simulink model "lab3_ssEvals"  (R2024b)
settings: Solver=VariableStepAuto  StartTime=0.0  StopTime=sIn.simulation_time  RelTol=1e-3
undefined symbols (not defined in the file or in its folder): feedback, filt, sens
libraries: simulink x1
settings Model: Creator=pries  LastModifiedBy=pries
settings DataIOCC: ReturnWorkspaceOutputs=off

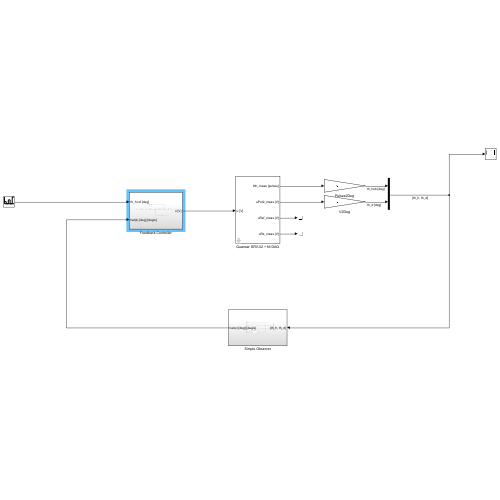
[thumbnail: Simulink's stored preview of the top-level diagram]
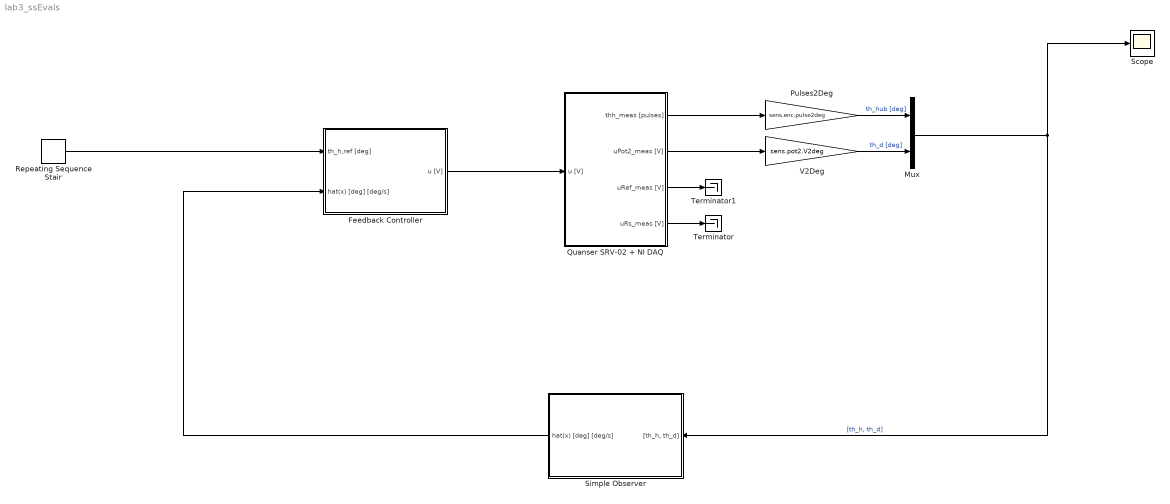
== system lab3_ssEvals ==
  Feedback Controller : Subsystem
  Mux : Mux  Inputs=2
  Pulses2Deg : Gain  Gain=sens.enc.pulse2deg
  Quanser SRV-02 + NI DAQ : Subsystem  mask(Quanser SRV-02 (with resonant load) + NI DAQ){Ts=0.001, fricType=Coulomb + viscous, lockShaft=off, beamInitPos=10}
      mask prompts: Ts "NI DAQ Sample Time:"; fricType "Friction model"; lockShaft "Lock motor shaft"; beamInitPos "Beam initial position [deg]:"
      mask help: Quanser SRV-02 (with resonant load) + NI DAQ model.
      mask init:
      | %%
      | % Riccardo Antonello (riccardo.antonello@unipd.it)
      | %
      | % April 28, 2020
      | %
      | % Dept. of Information Engineering, University of Padova
      | %
      | 
      | %%  Conversion gains
      | deg2rad = pi/180;                   %   [deg]   -> [rad]
      | rad2deg = 180/pi;                   %   [rad]   -> [deg]
      | 
      | 
      | %%  Sensors data
      | 
      | %   shunt resistor
      | sens.curr.Rs = 0.5;   
      | 
      | %   Hewlett-Packard HEDS-5540#A06 optical encoder
      | sens.enc.ppr = 500*4;                                                   %   pulses per rotation
      | sens.enc.pulse2deg = 360/sens.enc.ppr;                                  %   [pulses] -> [deg]
      | sens.enc.pulse2rad = 2*pi/sens.enc.ppr;                                 %   [pulses] -> [rad]
      | sens.enc.deg2pulse = sens.enc.ppr/360;                                  %   [deg] -> [pulses]
      | sens.enc.rad2pulse = sens.enc.ppr/2/pi;                                 %   [rad] -> [pulses]
      | 
      | %   potentiometer 2 (Spectrol 357-0-0-103) - installed on hub
      | sens.pot2.range.R      = 10e3;                                          %   ohmic value range 
      | sens.pot2.range.V      = 5;                                             %   voltage range
      | sens.pot2.range.th_deg = 340;                                           %   angle range [deg]
      | sens.pot2.range.th     = sens.pot2.range.th_deg * deg2rad;              %   angle range [rad]                           
      | sens.pot2.deg2V        = sens.pot2.range.V / sens.pot2.range.th_deg;    %   sensitivity [V/deg]
      | sens.pot2.rad2V        = sens.pot2.range.V / sens.pot2.range.th;        %   sensitivity [V/rad]
      | sens.pot2.V2deg        = 1/sens.pot2.deg2V;                             %   conversion gain [V] -> [deg]
      | sens.pot2.V2rad        = 1/sens.pot2.rad2V;                             %   conversion gain [V] -> [rad]
      | sens.pot2.noise.var    = 3.5e-7;                                        %   out noise variance [V^2]
      | 
      | 
      | %%  Data acquisition board (daq) data
      | 
      | %   NI PCI-6221 DAC data
      | daq.dac.bits = 16;                                  %   resolution (bits)
      | daq.dac.fs   = 10;                                  %   full scale 
      | daq.dac.q    = 2*daq.dac.fs/(2^daq.dac.bits-1);     %	quantization
      | 
      | %   NI PCI-6221 ADC data
      | daq.adc.bits = 16;                                  %   resolution (bits)
      | daq.adc.fs   = 10;                                  %   full scale (as set in SLDRT Analog Input block)
      | daq.adc.q    = 2*daq.adc.fs/(2^daq.adc.bits-1);     %   quantization   
      | 
      | 
      | %%  Set beam initial position
      | % SRV02Handle = find_system(gcb, ...
      | %     'LookUnderMasks', 'on', ...
      | %     'FindAll', 'on', ...
      | %     'FollowLinks', 'on', ...
      | %     'SearchDepth', '1', ...
      | %     'BlockType', 'ModelReference', ...
      | %     'Name', 'Quanser SRV-02');
      | %
      | % %get_param(SRV02Handle, 'InstanceParameters')
      | % InstanceParams = get_param(SRV02Handle, 'InstanceParameters');
      | % for k = 1:length(InstanceParams)
      | %     if strcmp(InstanceParams(k).Name, 'thb0')
      | %         if lockShaft
      | %             InstanceParams(k).Value = sprintf('%f', beamInitPos);
      | %         else
      | %             InstanceParams(k).Value = sprintf('%f', 0);    
      | %         end
      | %         set_param(SRV02Handle, 'InstanceParameters', InstanceParams);
      | %         break;
      | %     end
      | % end
      | 
      | if lockShaft
      |     thb0 = beamInitPos;
      | else
      |     thb0 = 0;    
      | end
      | 
      | 
      | %%  Mask initialization
      | if lockShaft
      |     
      |     %   find Inport handle
      |     InPortHandle = find_system(gcb, ...
      |         'LookUnderMasks', 'on', ...
      |         'FindAll', 'on', ...
      |         'FollowLinks', 'on', ...
      |         'SearchDepth', '1', ...
      |         'BlockType', 'Inport', ...
      |         'Name', 'u [V]');
      |     
      |     if ~isempty(InPortHandle)
      |     
      |         %   find DAC handle
      |         DACHandle = find_system(gcb, ...
      |             'LookUnderMasks', 'on', ...
      |             'FindAll', 'on', ...
      |             'FollowLinks', 'on', ...
      |             'SearchDepth', '1', ...
      |             'BlockType', 'SubSystem', ...
      |             'Name', 'DAC');  
      | 
      |         %   remove Inport output connection   
      |         InportConn = get_param(InPortHandle, 'PortConnectivity');
      |         delete_line(gcb, InportConn.Position);
      | 
      |         %   remove Inport block
      |         delete_block(InPortHandle);
      | 
      |         %   add Constant block
      |         ConstantHandle = add_block( ...
      |             'simulink/Sources/Constant', [gcb, '/u [V]'], ...
      |             'Position', [20   -37    50   -23], ...
      |             'Value', '0');
      | 
      |         %   connect Constant to DAC block
      |         DACPortHandles = get_param(DACHandle, 'PortHandles');
      |         ConstantPortHandles = get_param(ConstantHandle, 'PortHandles');
      |         add_line(gcb, ConstantPortHandles.Outport(1), DACPortHandles.Inport(1));
      |     
      |     end
      |     
      | else
      |     
      |     %   find Constant handle
      |     ConstantHandle = find_system(gcb, ...
      |         'LookUnderMasks', 'on', ...
      |         'FindAll', 'on', ...
      |         'FollowLinks', 'on', ...
      |         'SearchDepth', '1', ...
      |         'BlockType', 'Constant', ...
      |         'Name', 'u [V]');
      |     
      |     if ~isempty(ConstantHandle)
      |     
      |         %   find DAC handle
      |         DACHandle = find_system(gcb, ...
      |             'LookUnderMasks', 'on', ...
      |             'FindAll', 'on', ...
      |             'FollowLinks', 'on', ...
      |             'SearchDepth', '1', ...
      |             'BlockType', 'SubSystem', ...
      |             'Name', 'DAC');  
      |  
      |         %   remove Constant output connection   
      |         ConstantConn = get_param(ConstantHandle, 'PortConnectivity');
      |         delete_line(gcb, ConstantConn.Position);
      | 
      |         %   remove Inport block
      |         delete_block(ConstantHandle);   
      | 
      |         %   add Inport block
      |         InportHandle = add_block( ...
      |             'simulink/Sources/In1', [gcb, '/u [V]'], ...
      |             'Position', [20   -37    50   -23], ...
      |             'Port', '1');
      | 
      |         %   connect Constant to DAC block
      |         DACPortHandles = get_param(DACHandle, 'PortHandles');
      |         InportPortHandles = get_param(InportHandle, 'PortHandles');
      |         add_line(gcb, InportPortHandles.Outport(1), DACPortHandles.Inport(1));
      |     
      |      end
      |     
      | end
      mask Help:
      | Riccardo Antonello (antonello@dei.unipd.it)
      | 
      | April 28, 2020
      | 
      | Dept. of Information Engineering, University of Padova
      mask TypeOptions fricType: Coulomb + viscous | Karnopp
      mask Callback lockShaft:
      | %   get status of check box
      | lockShaft = get_param(gcb, 'lockShaft');
      | 
      | %   get current value of MaskVisibilities property
      | maskVisibilities = get_param(gcb, 'MaskVisibilities');
      | 
      | %   set visibility of the dialog box element
      | if strcmp(lockShaft, 'on')
      |     maskVisibilities{4} = 'on';
      | else
      |     maskVisibilities{4} = 'off';
      | end
      | 
      | % Set the 'MaskVisibilities' property for each parameter in mask
      | set_param( gcb, 'MaskVisibilities', maskVisibilities);
  Repeating Sequence Stair : simulink/Sources/Repeating Sequence Stair  OutValues=sIn.position  tsamp=sIn.step_time  OutMin=[]  OutMax=[]  OutDataTypeStr=double  OutputDataTypeScalingMode=double  OutDataType=fixdt(0,8)  ConRadixGroup=Best Precision: Vector-wise  OutScaling=2^-12
  Scope : Scope
  Simple Observer : Subsystem
  Terminator : Terminator
  Terminator1 : Terminator
  V2Deg : Gain  Gain=sens.pot2.V2deg
  wires:
  Quanser SRV-02 + NI DAQ/1(thh_meas [pulses]) -> Pulses2Deg/1
  Quanser SRV-02 + NI DAQ/2(uPot2_meas [V]) -> V2Deg/1
  Quanser SRV-02 + NI DAQ/4(uRs_meas [V]) -> Terminator/1
  Quanser SRV-02 + NI DAQ/3(uRef_meas [V]) -> Terminator1/1
  Pulses2Deg/1 -> Mux/1  "th_hub [deg]"
  V2Deg/1 -> Mux/2  "th_d [deg]"
  Mux/1 -> Simple Observer/1("[th_h, th_d]"), Scope/1  "[th_h, th_d]"
  Feedback Controller/1(u [V]) -> Quanser SRV-02 + NI DAQ/1(u [V])
  Simple Observer/1(hat(x) [deg] [deg/s]) -> Feedback Controller/2(hat(x) [deg] [deg/s])
  Repeating Sequence Stair/1 -> Feedback Controller/1(th_h,ref [deg])

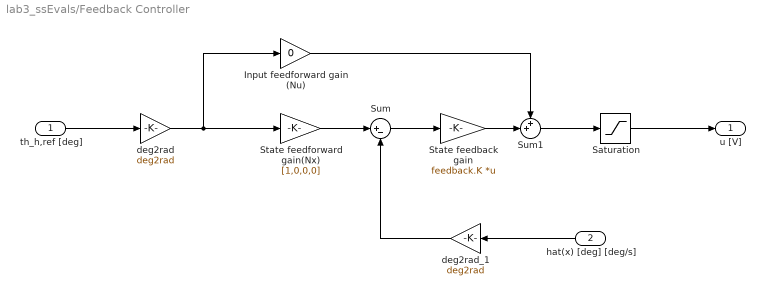
== system lab3_ssEvals/Feedback Controller ==
  th_h,ref [deg] : Inport
  hat(x) [deg] [deg/s] : Inport  Port=2
  Input feedforward gain (Nu) : Gain  Gain=0
  Saturation : Saturate  UpperLimit=10  LowerLimit=-10
  State feedback gain : Gain  Gain=feedback.K  Multiplication=Matrix(K*u)
  State feedforward gain(Nx) : Gain  Gain=[1,0,0,0]
  Sum : Sum  Inputs=|+-
  Sum1 : Sum  Inputs=++|
  deg2rad : Gain  Gain=deg2rad
  deg2rad_1 : Gain  Gain=deg2rad
  u [V] : Outport
  wires:
  deg2rad_1/1 -> Sum/2
  Input feedforward gain (Nu)/1 -> Sum1/1
  State feedback gain/1 -> Sum1/2
  Sum1/1 -> Saturation/1
  Sum/1 -> State feedback gain/1
  Saturation/1 -> u [V]/1
  State feedforward gain(Nx)/1 -> Sum/1
  deg2rad/1 -> State feedforward gain(Nx)/1, Input feedforward gain (Nu)/1
  th_h,ref [deg]/1 -> deg2rad/1
  hat(x) [deg] [deg/s]/1 -> deg2rad_1/1

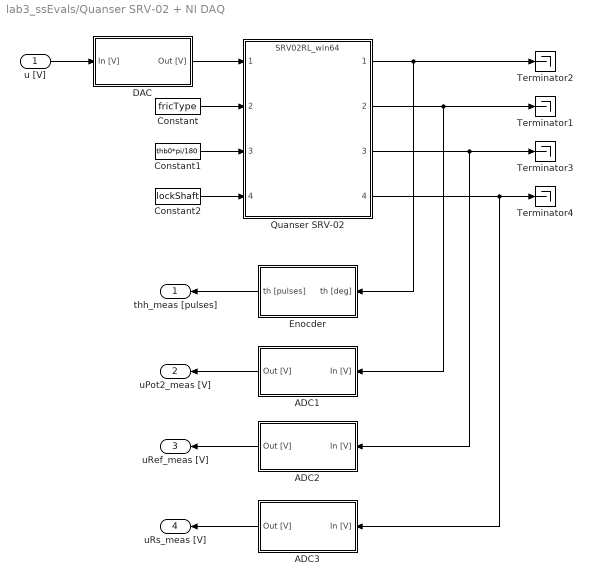
== system lab3_ssEvals/Quanser SRV-02 + NI DAQ ==
  u [V] : Inport
  ADC1 : Subsystem
  ADC2 : Subsystem
  ADC3 : Subsystem
  Constant : Constant  Value=fricType
  Constant1 : Constant  Value=thb0*pi/180  SampleTime=Inf
  Constant2 : Constant  Value=lockShaft  SampleTime=Inf
  DAC : Subsystem
  Enocder : Subsystem
  Quanser SRV-02 : ModelReference  ModelNameDialog=SRV02RL_win64.slxp  ModelReferenceVersion=1.76  CopyOfModelProtected=on
  Terminator{1..4} (4 alike) : Terminator
  thh_meas [pulses] : Outport
  uPot2_meas [V] : Outport  Port=2
  uRef_meas [V] : Outport  Port=3
  uRs_meas [V] : Outport  Port=4
  wires:
  u [V]/1 -> DAC/1(In [V])
  ADC2/1(Out [V]) -> uRef_meas [V]/1
  Quanser SRV-02/4 -> Terminator4/1, ADC3/1(In [V])
  Constant2/1 -> Quanser SRV-02/4
  Constant1/1 -> Quanser SRV-02/3
  ADC1/1(Out [V]) -> uPot2_meas [V]/1
  Quanser SRV-02/3 -> Terminator3/1, ADC2/1(In [V])
  Constant/1 -> Quanser SRV-02/2
  Quanser SRV-02/1 -> Enocder/1(th [deg]), Terminator2/1
  Quanser SRV-02/2 -> Terminator1/1, ADC1/1(In [V])
  DAC/1(Out [V]) -> Quanser SRV-02/1
  ADC3/1(Out [V]) -> uRs_meas [V]/1
  Enocder/1(th [pulses]) -> thh_meas [pulses]/1

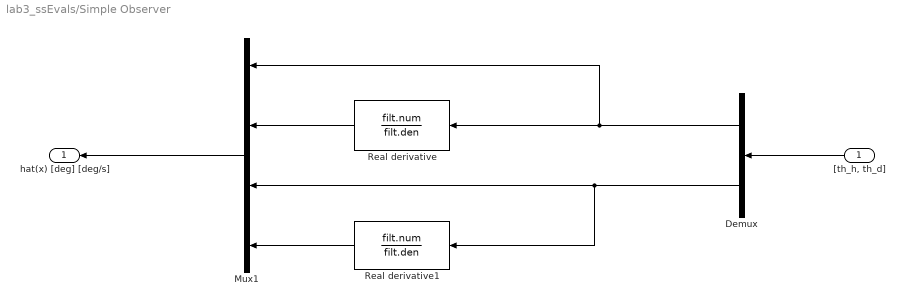
== system lab3_ssEvals/Simple Observer ==
  "[th_h, th_d]" : Inport
  Demux : Demux  Outputs=2
  Mux1 : Mux
  Real derivative : TransferFcn  Numerator=filt.num  Denominator=filt.den
  Real derivative1 : TransferFcn  Numerator=filt.num  Denominator=filt.den
  hat(x) [deg] [deg/s] : Outport
  wires:
  Demux/1 -> Mux1/1, Real derivative/1
  Demux/2 -> Mux1/3, Real derivative1/1
  Real derivative/1 -> Mux1/2
  Mux1/1 -> hat(x) [deg] [deg/s]/1
  Real derivative1/1 -> Mux1/4
  "[th_h, th_d]"/1 -> Demux/1

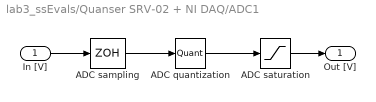
== system lab3_ssEvals/Quanser SRV-02 + NI DAQ/ADC1 ==
  In [V] : Inport
  ADC quantization : Quantizer  QuantizationInterval=daq.adc.q
  ADC sampling : ZeroOrderHold  SampleTime=Ts
  ADC saturation : Saturate  UpperLimit=daq.adc.fs  LowerLimit=-daq.adc.fs
  Out [V] : Outport
  wires:
  ADC quantization/1 -> ADC saturation/1
  In [V]/1 -> ADC sampling/1
  ADC sampling/1 -> ADC quantization/1
  ADC saturation/1 -> Out [V]/1

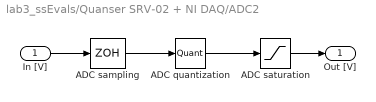
== system lab3_ssEvals/Quanser SRV-02 + NI DAQ/ADC2 ==
  In [V] : Inport
  ADC quantization : Quantizer  QuantizationInterval=daq.adc.q
  ADC sampling : ZeroOrderHold  SampleTime=Ts
  ADC saturation : Saturate  UpperLimit=daq.adc.fs  LowerLimit=-daq.adc.fs
  Out [V] : Outport
  wires:
  ADC saturation/1 -> Out [V]/1
  ADC sampling/1 -> ADC quantization/1
  In [V]/1 -> ADC sampling/1
  ADC quantization/1 -> ADC saturation/1

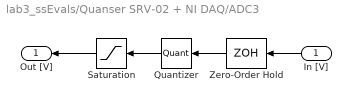
== system lab3_ssEvals/Quanser SRV-02 + NI DAQ/ADC3 ==
  In [V] : Inport
  Quantizer : Quantizer  QuantizationInterval=daq.adc.q
  Saturation : Saturate  UpperLimit=daq.adc.fs  LowerLimit=-daq.adc.fs
  Zero-Order Hold : ZeroOrderHold  SampleTime=Ts
  Out [V] : Outport
  wires:
  Zero-Order Hold/1 -> Quantizer/1
  Quantizer/1 -> Saturation/1
  In [V]/1 -> Zero-Order Hold/1
  Saturation/1 -> Out [V]/1

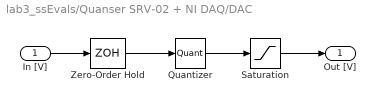
== system lab3_ssEvals/Quanser SRV-02 + NI DAQ/DAC ==
  In [V] : Inport
  Quantizer : Quantizer  QuantizationInterval=daq.dac.q
  Saturation : Saturate  UpperLimit=daq.dac.fs  LowerLimit=-daq.dac.fs
  Zero-Order Hold : ZeroOrderHold  SampleTime=Ts
  Out [V] : Outport
  wires:
  Saturation/1 -> Out [V]/1
  Zero-Order Hold/1 -> Quantizer/1
  In [V]/1 -> Zero-Order Hold/1
  Quantizer/1 -> Saturation/1

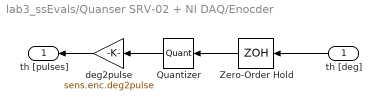
== system lab3_ssEvals/Quanser SRV-02 + NI DAQ/Enocder ==
  th [deg] : Inport
  Quantizer : Quantizer  QuantizationInterval=sens.enc.pulse2deg
  Zero-Order Hold : ZeroOrderHold  SampleTime=Ts
  deg2pulse : Gain  Gain=sens.enc.deg2pulse
  th [pulses] : Outport
  wires:
  deg2pulse/1 -> th [pulses]/1
  Zero-Order Hold/1 -> Quantizer/1
  th [deg]/1 -> Zero-Order Hold/1
  Quantizer/1 -> deg2pulse/1
